simulink model "fismodel"  (R2023a)
settings: Solver=VariableStepAuto  StartTime=0.0  StopTime=10.0  RelTol=1e-3
libraries: fuzblock x1
settings Model: Creator=aymanouchker  LastModifiedBy=aymanouchker

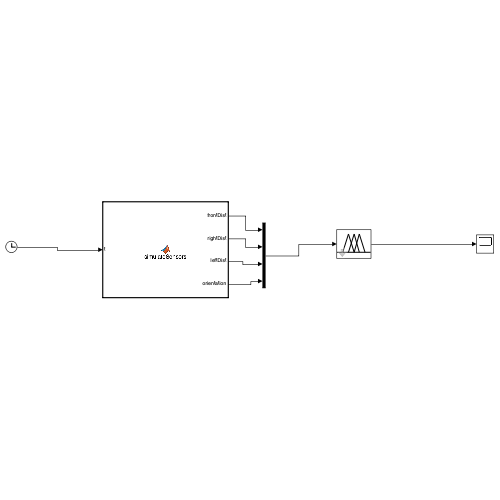
[thumbnail: Simulink's stored preview of the top-level diagram]
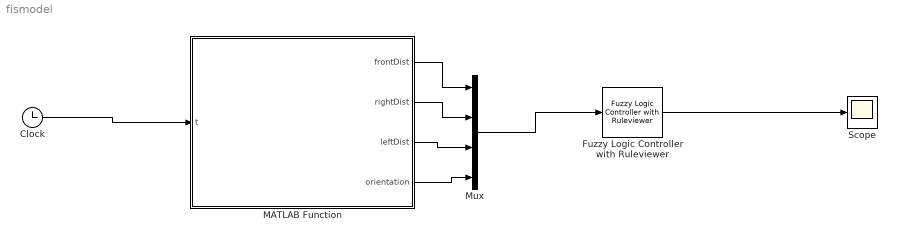
== system fismodel ==
  Clock : Clock
  Fuzzy Logic Controller with Ruleviewer : fuzblock/Fuzzy Logic  Controller  with Ruleviewer  fismatrix=robot_navigation_fis  Ts=2
  MATLAB Function : MATLAB Function  TreatAsAtomicUnit=on
  Mux : Mux
  Scope : Scope
  wires:
  Fuzzy Logic Controller with Ruleviewer/1 -> Scope/1
  Mux/1 -> Fuzzy Logic Controller with Ruleviewer/1
  MATLAB Function/3(leftDist) -> Mux/3
  MATLAB Function/2(rightDist) -> Mux/2
  MATLAB Function/1(frontDist) -> Mux/1
  MATLAB Function/4(orientation) -> Mux/4
  Clock/1 -> MATLAB Function/1(t)

== matlab function fismodel/MATLAB Function ==
  data: t input; frontDist output; rightDist output; leftDist output; orientation output
function [frontDist, rightDist, leftDist, orientation] = simulateSensors(t)
    % Simulate dynamic sensor readings
    frontDist = 50 + 30*sin(t); % Example: distance varies with time
    rightDist = 50 + 30*sin(t + pi/2);
    leftDist = 50 + 30*sin(t + pi);
    orientation = mod(t * 30, 360); % Example: orientation changes linearly with time
end
